simulink model "TPTC_Vehicle_dynamics_pedal2torque_NeglectSOC"  (R2026a)
settings: Solver=ode23tb  StopTime=40
model workspace (MAT data in the model file):
  BattChrgMax = -500000
  BattDischrgMax = 500000
  ChrgLmt_bpt = [1 1 1 1 1 1 1 1 0.7 0.35 0]
  DischrgLmt_bpt = [0 0.35 0.7 1 1 1 1 1 1 1 1]
  SOC_bpt = [0 10 20 30 40 50 60 70 80 90 100]
  motorMaxTorqueNm = [500 500 500 500 500 500 416.666666667 357.142857143 312.5 277.777777778 250 227.272727273 ... (16 elements, 1x16)]
  motorSpeedRadPs = [0 40 80 120 160 200 240 280 320 360 400 440 ... (16 elements, 1x16)]
values from neighbouring files (symbols this model uses):
  alpha_thr = Simulink.Parameter(300)    [init_MCU_ASR_params_only.m]
  eta_drv = Simulink.Parameter(0.95)    [init_MCU_ASR_params_only.m]
  gear_ratio_F = Simulink.Parameter(10.91)    [init_MCU_ASR_params_only.m]
  gear_ratio_R = Simulink.Parameter(11.62)    [init_MCU_ASR_params_only.m]
  J_axle = Simulink.Parameter(2*I_tire)    [init_MCU_ASR_params_only.m]
  Kd_damp = Simulink.Parameter(0.025)    [init_MCU_ASR_params_only.m]
  R_tire = Simulink.Parameter(r)    [init_MCU_ASR_params_only.m]
  T_active = Simulink.Parameter(15)    [init_MCU_ASR_params_only.m]
  T_damp_lim = Simulink.Parameter(18)    [init_MCU_ASR_params_only.m]
  tau_lpf_damp = Simulink.Parameter(0.060)    [init_MCU_ASR_params_only.m]
  Tlim_down_rate = Simulink.Parameter(2000)    [init_MCU_ASR_params_only.m]
  Tlim_up_rate = Simulink.Parameter(120)    [init_MCU_ASR_params_only.m]
  Tlim_warn_rate = Simulink.Parameter(600)    [init_MCU_ASR_params_only.m]
  Tmax_mot = Simulink.Parameter(Tn_motor)    [init_MCU_ASR_params_only.m]
  Ts_asr = Simulink.Parameter(0.001)    [init_MCU_ASR_params_only.m]
undefined symbols (not defined in the file or in its folder): dspblkCoreblockFVToolHelper, gcbh, gear_ratio
libraries: autolibsharedcoupling x8, simulink x3, autolibshareddiff x2, autolibmappedmotor x2, slpidlib x1, autolibdatasheetbattery x1, sim3dlib x1, sim3dautolib x1, vehdynlibsteering x1
(part 3 of 4)

== matlab function TPTC_Vehicle_dynamics_pedal2torque_NeglectSOC/03_MCU_ASR_Controller1/Slip_Detector_Rear/MATLAB Function ==
  data: Te input; risk output; warn output; alpha input; Tload input; omega input; Te_opp input; alpha_opp input; Tload_opp input; omega_opp input; T_active input; state output; alpha_thr input; Ts input; load_ratio output; follow_bad output; axis_diverge output; startup_guard output
function [risk,warn,state,load_ratio,follow_bad,axis_diverge,startup_guard] = f( ...
    Te,alpha,Tload,omega, ...
    Te_opp,alpha_opp,Tload_opp,omega_opp, ...
    T_active,alpha_thr,Ts)
%#codegen

% ============================================================
% MCU级 TCPC/ASR Slip Detector
%
% 核心判据：
% 1. Tload_est / Te 偏低
% 2. Te 增加时，Tload_est 不跟随增加
% 3. alpha 异常升高作为确认条件
%
% axis_diverge 只做诊断输出，不单独触发 warn/risk
%
% state:
%   0 Normal
%   1 Warning
%   2 Risk
% ============================================================

persistent risk_z warn_z
persistent Te_z Tload_z omega_z omega_opp_z
persistent active_cnt risk_enter_cnt warn_enter_cnt risk_exit_cnt warn_exit_cnt

if isempty(risk_z)
    risk_z = false;
    warn_z = false;

    Te_z = 0.0;
    Tload_z = 0.0;
    omega_z = 0.0;
    omega_opp_z = 0.0;

    active_cnt = 0.0;
    risk_enter_cnt = 0.0;
    warn_enter_cnt = 0.0;
    risk_exit_cnt = 0.0;
    warn_exit_cnt = 0.0;
end

% =========================
% 采样时间保护
% =========================
if Ts <= 0.0
    Ts_eff = 1e-3;
else
    Ts_eff = Ts;
end

% =========================
% 可标定参数
% =========================

% 负载比例阈值
k_load_risk = 0.72;
k_load_warn = 0.86;

% 跟随性阈值
k_follow_risk = 0.20;
k_follow_warn = 0.40;

% alpha 阈值
alpha_warn_gain = 0.65;
alpha_risk_gain = 1.00;

% 起步保护
startup_guard_time = 0.30;
startup_guard_steps = ceil(startup_guard_time / Ts_eff);

% 起步阶段只允许较强 risk
alpha_start_risk_gain = 1.40;
k_load_start_risk = 0.55;

% 进入确认时间
% risk 不要太慢，否则压不住滑移；warn 稍微确认
risk_enter_confirm_time = 0.005;  % 5 ms
warn_enter_confirm_time = 0.020;  % 20 ms

risk_enter_steps = ceil(risk_enter_confirm_time / Ts_eff);
warn_enter_steps = ceil(warn_enter_confirm_time / Ts_eff);

% 退出确认时间
risk_exit_confirm_time = 0.080;   % 80 ms，避免频繁退出
warn_exit_confirm_time = 0.050;   % 50 ms

risk_exit_steps = ceil(risk_exit_confirm_time / Ts_eff);
warn_exit_steps = ceil(warn_exit_confirm_time / Ts_eff);

% dTe 太小时不判断跟随性
dTe_min = max(0.02*T_active, 0.5);

% 前后轴分化诊断阈值
alpha_diff_thr = 0.80*alpha_thr;
omega_diff_thr = 5.0;
omega_diff_rate_thr = 50.0;

% =========================
% 有效驱动区
% =========================
active = (Te > T_active);

if active
    active_cnt = active_cnt + 1.0;
else
    active_cnt = 0.0;
end

startup_guard = active && (active_cnt <= startup_guard_steps);

% =========================
% 负载比例
% =========================
Te_eff = max(Te, 1.0);
load_ratio_raw = Tload / Te_eff;

if load_ratio_raw < 0.0
    load_ratio = 0.0;
elseif load_ratio_raw > 2.0
    load_ratio = 2.0;
else
    load_ratio = load_ratio_raw;
end

load_gap_risk = (load_ratio < k_load_risk);
load_gap_warn = (load_ratio < k_load_warn);

% =========================
% Tload 是否随 Te 增加
% =========================
dTe = Te - Te_z;
dTload = Tload - Tload_z;

torque_rising = (dTe > dTe_min);

follow_bad_risk = torque_rising && (dTload < k_follow_risk*dTe);
follow_bad_warn = torque_rising && (dTload < k_follow_warn*dTe);

follow_bad = follow_bad_risk;

% =========================
% alpha 异常
% =========================
alpha_risk = (alpha > alpha_risk_gain*alpha_thr);
alpha_warn = (alpha > alpha_warn_gain*alpha_thr);

% =========================
% 前后轴分化，仅诊断
% =========================
omega_diff = omega - omega_opp;
omega_diff_z = omega_z - omega_opp_z;
d_omega_diff = (omega_diff - omega_diff_z) / Ts_eff;

alpha_diverge = (alpha > alpha_opp + alpha_diff_thr) && alpha_warn;

omega_diverge = (~startup_guard) && ...
                (omega_diff > omega_diff_thr) && ...
                (d_omega_diff > omega_diff_rate_thr);

axis_diverge = alpha_diverge || omega_diverge;

% =========================
% 原始进入判据
% =========================
if startup_guard

    % 起步保护阶段：
    % 不允许 warn，只允许强 risk
    warn_enter_raw = false;

    risk_enter_raw = active && ...
                     (alpha > alpha_start_risk_gain*alpha_thr) && ...
                     ((load_ratio < k_load_start_risk) || follow_bad_risk);

else

    % 正常阶段：
    % axis_diverge 不直接触发
    risk_enter_raw = active && ...
                     alpha_risk && ...
                     (load_gap_risk || follow_bad_risk);

    warn_enter_raw = active && ...
                     alpha_warn && ...
                     (load_gap_warn || follow_bad_warn);
end

% =========================
% 进入确认
% =========================
if risk_enter_raw
    risk_enter_cnt = risk_enter_cnt + 1.0;
else
    risk_enter_cnt = 0.0;
end

if warn_enter_raw
    warn_enter_cnt = warn_enter_cnt + 1.0;
else
    warn_enter_cnt = 0.0;
end

risk_enter = (risk_enter_cnt >= risk_enter_steps);
warn_enter = (warn_enter_cnt >= warn_enter_steps);

% =========================
% 退出判据
% =========================
risk_exit_raw = (~active) || ...
                ( ...
                  (alpha < 0.45*alpha_thr) && ...
                  (load_ratio > 0.88) && ...
                  (~follow_bad_warn) ...
                );

warn_exit_raw = (~active) || ...
                ( ...
                  (alpha < 0.35*alpha_thr) && ...
                  (load_ratio > 0.96) && ...
                  (~follow_bad_warn) ...
                );

if risk_exit_raw
    risk_exit_cnt = risk_exit_cnt + 1.0;
else
    risk_exit_cnt = 0.0;
end

if warn_exit_raw
    warn_exit_cnt = warn_exit_cnt + 1.0;
else
    warn_exit_cnt = 0.0;
end

risk_exit = (risk_exit_cnt >= risk_exit_steps);
warn_exit = (warn_exit_cnt >= warn_exit_steps);

% =========================
% risk 滞回
% =========================
if risk_z
    if risk_exit
        risk_z = false;
        risk_exit_cnt = 0.0;
    end
else
    if risk_enter
        risk_z = true;
        risk_enter_cnt = 0.0;
    end
end

% =========================
% warn 滞回
% =========================
if risk_z
    warn_z = false;
    warn_exit_cnt = 0.0;
else
    if warn_z
        if warn_exit
            warn_z = false;
            warn_exit_cnt = 0.0;
        end
    else
        if warn_enter
            warn_z = true;
            warn_enter_cnt = 0.0;
        end
    end
end

% =========================
% 输出
% =========================
risk = risk_z;
warn = warn_z;

if risk_z
    state = 2.0;
elseif warn_z
    state = 1.0;
else
    state = 0.0;
end

% =========================
% 更新历史量
% =========================
Te_z = Te;
Tload_z = Tload;
omega_z = omega;
omega_opp_z = omega_opp;

end

== matlab function TPTC_Vehicle_dynamics_pedal2torque_NeglectSOC/03_MCU_ASR_Controller1/Torque_Limiter_Front/Fast_Down_Slow_Up_Limiter ==
  data: T_vcu input; Tlim output; risk input; warn input; Tload input; Tmax_mot parameter; state output; Tlim_up_rate parameter; Tlim_down_rate parameter; Tlim_warn_rate parameter; Ts_asr parameter
function [Tlim,state] = f(T_vcu,risk,warn,Tload,Tmax_mot,Tlim_up_rate,Tlim_down_rate,Tlim_warn_rate,Ts_asr)
%#codegen

% ============================================================
% MCU级 TCPC/ASR 限扭器 v5
%
% state:
%   0 Normal
%   1 Warning
%   2 SpinDown
%   3 Hold
%   4 Recovery
%
% 核心策略：
%   1. risk 时快速降低 Tcap 和 Tlim
%   2. 打滑后进入 Hold，不立即恢复
%   3. Recovery 只恢复到 Tcap
%   4. Tcap 只在稳定后小斜率上探
%   5. 避免恢复-打滑-恢复的大幅搏动
% ============================================================

persistent Tlim_z state_z hold_cnt recover_cnt drive_cnt
persistent Tload_lpf_z first_run
persistent Tcap_z stable_cnt

if isempty(Tlim_z)
    Tlim_z = 0.0;
    state_z = 0.0;
    hold_cnt = 0.0;
    recover_cnt = 0.0;
    drive_cnt = 0.0;

    Tload_lpf_z = 0.0;
    first_run = true;

    Tcap_z = 0.0;
    stable_cnt = 0.0;
end

% =========================
% 状态定义
% =========================
S_NORMAL   = 0.0;
S_WARNING  = 1.0;
S_SPINDOWN = 2.0;
S_HOLD     = 3.0;
S_RECOVERY = 4.0;

% =========================
% 采样时间保护
% =========================
if Ts_asr <= 0.0
    Ts = 1e-3;
else
    Ts = Ts_asr;
end

% =========================
% 可标定参数
% =========================

% 状态时间
spin_hold_time = 0.25;        % 低扭矩保持 250 ms
recovery_min_time = 0.35;     % Recovery 至少 350 ms

spin_hold_steps = ceil(spin_hold_time / Ts);
recovery_min_steps = ceil(recovery_min_time / Ts);

% Tload 低通
tau_Tload = 0.060;            % 60 ms

% SpinDown 目标
T_decel_margin = 18.0;        % T_spin_target = Tload_ref - margin
T_spin_min = 0.0;
T_spin_keep_min = 0.0;

% 动态 Tcap
Tcap_margin_recover = 8.0;    % risk 后 Tcap 收敛到 Tload_ref + 8
Tcap_drop_rate = 5000.0;      % risk 时 Tcap 下降速率
Tcap_min = 0.0;

% Tcap 试探增长
Tcap_probe_rate_slow = 6.0;   % 低附着/不确定
Tcap_probe_rate_mid  = 25.0;  % 中等
Tcap_probe_rate_fast = 80.0;  % 高附着确认

stable_time_for_probe = 0.30; % 稳定 300 ms 后才允许 Tcap 上探
stable_steps_for_probe = ceil(stable_time_for_probe / Ts);

% warn 处理
warn_freeze_time = 0.10;      % Recovery 中 warn 冻结 100 ms
T_warn_min = 15.0;

% 上升速率
Tlim_normal_up_rate = 1.2*Tlim_up_rate;
Tlim_recovery_up_rate = 0.45*Tlim_up_rate;

% 起步软限制
startup_time = 0.60;
startup_steps = ceil(startup_time / Ts);
T_cmd_active_thr = max(1.0,0.02*Tmax_mot);
startup_ramp_rate = 0.40*Tmax_mot / max(startup_time,Ts);

% 最终输出斜率保护
Tlim_final_down_rate = max(Tlim_down_rate,1500.0);
Tlim_final_up_rate   = max(Tlim_recovery_up_rate,1.0);

% =========================
% 目标扭矩
% =========================
target_raw = min(max(T_vcu,0.0),Tmax_mot);

if first_run
    Tlim_z = 0.0;
    Tload_lpf_z = max(Tload,0.0);
    Tcap_z = target_raw;
    first_run = false;
end

% =========================
% 驱动计时
% =========================
cmd_active = target_raw > T_cmd_active_thr;

if cmd_active
    drive_cnt = drive_cnt + 1.0;
else
    drive_cnt = 0.0;
end

startup_phase = cmd_active && (drive_cnt <= startup_steps);

% =========================
% Tload 低通
% =========================
Tload_eff = Tload;

if Tload_eff < 0.0
    Tload_eff = 0.0;
end

a_lpf = Ts / (tau_Tload + Ts);
Tload_lpf_z = Tload_lpf_z + a_lpf*(Tload_eff - Tload_lpf_z);

Tload_ref = Tload_lpf_z;

% =========================
% Tcap 更新
% =========================

% 当前负载跟随程度
Tlim_eff = max(Tlim_z,1.0);
load_ratio_cap = Tload_ref / Tlim_eff;

load_follow_good = (load_ratio_cap > 0.90);
load_follow_mid  = (load_ratio_cap > 0.75);

if risk

    % risk 时快速压低 Tcap
    Tcap_target_down = Tload_ref + Tcap_margin_recover;

    if Tcap_target_down < Tcap_min
        Tcap_target_down = Tcap_min;
    end

    if Tcap_z > Tcap_target_down
        Tcap_z = Tcap_z - Tcap_drop_rate*Ts;

        if Tcap_z < Tcap_target_down
            Tcap_z = Tcap_target_down;
        end
    else
        Tcap_z = Tcap_target_down;
    end

    stable_cnt = 0.0;

else

    if ~warn
        stable_cnt = stable_cnt + 1.0;
    else
        stable_cnt = 0.0;
    end

    if stable_cnt >= stable_steps_for_probe

        if load_follow_good
            Tcap_probe_rate_now = Tcap_probe_rate_fast;
        elseif load_follow_mid
            Tcap_probe_rate_now = Tcap_probe_rate_mid;
        else
            Tcap_probe_rate_now = Tcap_probe_rate_slow;
        end

        if Tcap_z < target_raw
            Tcap_z = Tcap_z + Tcap_probe_rate_now*Ts;

            if Tcap_z > target_raw
                Tcap_z = target_raw;
            end
        else
            Tcap_z = target_raw;
        end
    end
end

% Tcap 限幅
if Tcap_z > Tmax_mot
    Tcap_z = Tmax_mot;
elseif Tcap_z < 0.0
    Tcap_z = 0.0;
end

% 实际目标被 Tcap 限制
target = min(target_raw,Tcap_z);

% VCU 请求降低时，立即跟随
if Tlim_z > target_raw
    Tlim_z = target_raw;
end

% =========================
% SpinDown 目标
% =========================
T_spin_target = Tload_ref - T_decel_margin;

if T_spin_target < T_spin_min
    T_spin_target = T_spin_min;
end

if T_spin_target > target_raw
    T_spin_target = target_raw;
end

T_spin_keep_eff = min(T_spin_keep_min,target_raw);
T_warn_min_eff = min(T_warn_min,target_raw);

% =========================
% 状态转移
% =========================
switch state_z

    case S_NORMAL

        hold_cnt = 0.0;
        recover_cnt = 0.0;

        if risk
            state_z = S_SPINDOWN;
            hold_cnt = spin_hold_steps;

        elseif warn
            state_z = S_WARNING;

        else
            state_z = S_NORMAL;
        end

    case S_WARNING

        if risk
            state_z = S_SPINDOWN;
            hold_cnt = spin_hold_steps;

        elseif warn
            state_z = S_WARNING;

        else
            if Tlim_z < target
                state_z = S_RECOVERY;
                recover_cnt = recovery_min_steps;
            else
                state_z = S_NORMAL;
            end
        end

    case S_SPINDOWN

        if risk
            state_z = S_SPINDOWN;
            hold_cnt = spin_hold_steps;
        else
            state_z = S_HOLD;
            hold_cnt = spin_hold_steps;
        end

    case S_HOLD

        if risk
            state_z = S_SPINDOWN;
            hold_cnt = spin_hold_steps;
        else
            if hold_cnt > 0.0
                hold_cnt = hold_cnt - 1.0;
                state_z = S_HOLD;
            else
                state_z = S_RECOVERY;
                recover_cnt = recovery_min_steps;
            end
        end

    case S_RECOVERY

        if risk
            state_z = S_SPINDOWN;
            hold_cnt = spin_hold_steps;

        elseif warn
            % warn 时只冻结，不强降
            state_z = S_HOLD;
            hold_cnt = ceil(warn_freeze_time / Ts);

        else
            if recover_cnt > 0.0
                recover_cnt = recover_cnt - 1.0;
                state_z = S_RECOVERY;
            else
                if Tlim_z < target
                    state_z = S_RECOVERY;
                else
                    state_z = S_NORMAL;
                    recover_cnt = 0.0;
                end
            end
        end

    otherwise

        state_z = S_NORMAL;
        hold_cnt = 0.0;
        recover_cnt = 0.0;
end

% =========================
% 计算 Tlim_ref
% =========================
Tlim_ref = Tlim_z;

if state_z == S_SPINDOWN

    % 快速降到 Tload_ref - margin
    if Tlim_z > T_spin_target
        Tlim_ref = Tlim_z - Tlim_down_rate*Ts;

        if Tlim_ref < T_spin_target
            Tlim_ref = T_spin_target;
        end
    else
        Tlim_ref = Tlim_z;
    end

    if Tlim_ref < T_spin_keep_eff
        Tlim_ref = T_spin_keep_eff;
    end

elseif state_z == S_HOLD

    % Hold：保持低扭矩；如果仍偏高，继续缓慢向 T_spin_target 靠近
    if Tlim_z > T_spin_target
        Tlim_ref = Tlim_z - 0.20*Tlim_down_rate*Ts;

        if Tlim_ref < T_spin_target
            Tlim_ref = T_spin_target;
        end
    else
        Tlim_ref = Tlim_z;
    end

    if Tlim_ref < T_spin_keep_eff
        Tlim_ref = T_spin_keep_eff;
    end

elseif state_z == S_WARNING

    % Warning：只轻微降扭
    Tlim_ref = Tlim_z - Tlim_warn_rate*Ts;

    if Tlim_ref < T_warn_min_eff
        Tlim_ref = T_warn_min_eff;
    end

    if Tlim_ref > target
        Tlim_ref = target;
    end

elseif state_z == S_RECOVERY

    % Recovery：只恢复到 target = min(T_vcu, Tcap)
    if target > Tlim_z
        Tlim_ref = Tlim_z + Tlim_recovery_up_rate*Ts;

        if Tlim_ref > target
            Tlim_ref = target;
        end
    else
        Tlim_ref = target;
    end

else

    % Normal：也只跟随 target = min(T_vcu, Tcap)
    if target > Tlim_z
        Tlim_ref = Tlim_z + Tlim_normal_up_rate*Ts;

        if Tlim_ref > target
            Tlim_ref = target;
        end
    else
        Tlim_ref = target;
    end
end

% =========================
% 起步软限制
% =========================
if startup_phase && ...
   (state_z == S_NORMAL || state_z == S_WARNING || state_z == S_RECOVERY)

    startup_Tlim = startup_ramp_rate * drive_cnt * Ts;

    if Tlim_ref > startup_Tlim
        Tlim_ref = startup_Tlim;
    end
end

% =========================
% 最终输出斜率保护
% =========================
dT = Tlim_ref - Tlim_z;

if dT > Tlim_final_up_rate*Ts
    dT = Tlim_final_up_rate*Ts;
elseif dT < -Tlim_final_down_rate*Ts
    dT = -Tlim_final_down_rate*Ts;
end

Tlim_z = Tlim_z + dT;

% =========================
% 最终限幅
% =========================
if Tlim_z > Tmax_mot
    Tlim_z = Tmax_mot;
elseif Tlim_z < 0.0
    Tlim_z = 0.0;
end

if Tlim_z > target_raw
    Tlim_z = target_raw;
end

Tlim = Tlim_z;
state = state_z;

end

== matlab function TPTC_Vehicle_dynamics_pedal2torque_NeglectSOC/03_MCU_ASR_Controller1/Torque_Limiter_Rear/Fast_Down_Slow_Up_Limiter ==
  data: T_vcu input; Tlim output; risk input; warn input; Tload input; state output; Tmax_mot parameter; Tlim_up_rate parameter; Tlim_down_rate parameter; Tlim_warn_rate parameter; Ts_asr parameter
function [Tlim,state] = f(T_vcu,risk,warn,Tload,Tmax_mot,Tlim_up_rate,Tlim_down_rate,Tlim_warn_rate,Ts_asr)
%#codegen

% ============================================================
% MCU级 TCPC/ASR 限扭器 v5
%
% state:
%   0 Normal
%   1 Warning
%   2 SpinDown
%   3 Hold
%   4 Recovery
%
% 核心策略：
%   1. risk 时快速降低 Tcap 和 Tlim
%   2. 打滑后进入 Hold，不立即恢复
%   3. Recovery 只恢复到 Tcap
%   4. Tcap 只在稳定后小斜率上探
%   5. 避免恢复-打滑-恢复的大幅搏动
% ============================================================

persistent Tlim_z state_z hold_cnt recover_cnt drive_cnt
persistent Tload_lpf_z first_run
persistent Tcap_z stable_cnt

if isempty(Tlim_z)
    Tlim_z = 0.0;
    state_z = 0.0;
    hold_cnt = 0.0;
    recover_cnt = 0.0;
    drive_cnt = 0.0;

    Tload_lpf_z = 0.0;
    first_run = true;

    Tcap_z = 0.0;
    stable_cnt = 0.0;
end

% =========================
% 状态定义
% =========================
S_NORMAL   = 0.0;
S_WARNING  = 1.0;
S_SPINDOWN = 2.0;
S_HOLD     = 3.0;
S_RECOVERY = 4.0;

% =========================
% 采样时间保护
% =========================
if Ts_asr <= 0.0
    Ts = 1e-3;
else
    Ts = Ts_asr;
end

% =========================
% 可标定参数
% =========================

% 状态时间
spin_hold_time = 0.25;        % 低扭矩保持 250 ms
recovery_min_time = 0.35;     % Recovery 至少 350 ms

spin_hold_steps = ceil(spin_hold_time / Ts);
recovery_min_steps = ceil(recovery_min_time / Ts);

% Tload 低通
tau_Tload = 0.060;            % 60 ms

% SpinDown 目标
T_decel_margin = 18.0;        % T_spin_target = Tload_ref - margin
T_spin_min = 0.0;
T_spin_keep_min = 0.0;

% 动态 Tcap
Tcap_margin_recover = 8.0;    % risk 后 Tcap 收敛到 Tload_ref + 8
Tcap_drop_rate = 5000.0;      % risk 时 Tcap 下降速率
Tcap_min = 0.0;

% Tcap 试探增长
Tcap_probe_rate_slow = 6.0;   % 低附着/不确定
Tcap_probe_rate_mid  = 25.0;  % 中等
Tcap_probe_rate_fast = 80.0;  % 高附着确认

stable_time_for_probe = 0.30; % 稳定 300 ms 后才允许 Tcap 上探
stable_steps_for_probe = ceil(stable_time_for_probe / Ts);

% warn 处理
warn_freeze_time = 0.10;      % Recovery 中 warn 冻结 100 ms
T_warn_min = 15.0;

% 上升速率
Tlim_normal_up_rate = 1.2*Tlim_up_rate;
Tlim_recovery_up_rate = 0.45*Tlim_up_rate;

% 起步软限制
startup_time = 0.60;
startup_steps = ceil(startup_time / Ts);
T_cmd_active_thr = max(1.0,0.02*Tmax_mot);
startup_ramp_rate = 0.40*Tmax_mot / max(startup_time,Ts);

% 最终输出斜率保护
Tlim_final_down_rate = max(Tlim_down_rate,1500.0);
Tlim_final_up_rate   = max(Tlim_recovery_up_rate,1.0);

% =========================
% 目标扭矩
% =========================
target_raw = min(max(T_vcu,0.0),Tmax_mot);

if first_run
    Tlim_z = 0.0;
    Tload_lpf_z = max(Tload,0.0);
    Tcap_z = target_raw;
    first_run = false;
end

% =========================
% 驱动计时
% =========================
cmd_active = target_raw > T_cmd_active_thr;

if cmd_active
    drive_cnt = drive_cnt + 1.0;
else
    drive_cnt = 0.0;
end

startup_phase = cmd_active && (drive_cnt <= startup_steps);

% =========================
% Tload 低通
% =========================
Tload_eff = Tload;

if Tload_eff < 0.0
    Tload_eff = 0.0;
end

a_lpf = Ts / (tau_Tload + Ts);
Tload_lpf_z = Tload_lpf_z + a_lpf*(Tload_eff - Tload_lpf_z);

Tload_ref = Tload_lpf_z;

% =========================
% Tcap 更新
% =========================

% 当前负载跟随程度
Tlim_eff = max(Tlim_z,1.0);
load_ratio_cap = Tload_ref / Tlim_eff;

load_follow_good = (load_ratio_cap > 0.90);
load_follow_mid  = (load_ratio_cap > 0.75);

if risk

    % risk 时快速压低 Tcap
    Tcap_target_down = Tload_ref + Tcap_margin_recover;

    if Tcap_target_down < Tcap_min
        Tcap_target_down = Tcap_min;
    end

    if Tcap_z > Tcap_target_down
        Tcap_z = Tcap_z - Tcap_drop_rate*Ts;

        if Tcap_z < Tcap_target_down
            Tcap_z = Tcap_target_down;
        end
    else
        Tcap_z = Tcap_target_down;
    end

    stable_cnt = 0.0;

else

    if ~warn
        stable_cnt = stable_cnt + 1.0;
    else
        stable_cnt = 0.0;
    end

    if stable_cnt >= stable_steps_for_probe

        if load_follow_good
            Tcap_probe_rate_now = Tcap_probe_rate_fast;
        elseif load_follow_mid
            Tcap_probe_rate_now = Tcap_probe_rate_mid;
        else
            Tcap_probe_rate_now = Tcap_probe_rate_slow;
        end

        if Tcap_z < target_raw
            Tcap_z = Tcap_z + Tcap_probe_rate_now*Ts;

            if Tcap_z > target_raw
                Tcap_z = target_raw;
            end
        else
            Tcap_z = target_raw;
        end
    end
end

% Tcap 限幅
if Tcap_z > Tmax_mot
    Tcap_z = Tmax_mot;
elseif Tcap_z < 0.0
    Tcap_z = 0.0;
end

% 实际目标被 Tcap 限制
target = min(target_raw,Tcap_z);

% VCU 请求降低时，立即跟随
if Tlim_z > target_raw
    Tlim_z = target_raw;
end

% =========================
% SpinDown 目标
% =========================
T_spin_target = Tload_ref - T_decel_margin;

if T_spin_target < T_spin_min
    T_spin_target = T_spin_min;
end

if T_spin_target > target_raw
    T_spin_target = target_raw;
end

T_spin_keep_eff = min(T_spin_keep_min,target_raw);
T_warn_min_eff = min(T_warn_min,target_raw);

% =========================
% 状态转移
% =========================
switch state_z

    case S_NORMAL

        hold_cnt = 0.0;
        recover_cnt = 0.0;

        if risk
            state_z = S_SPINDOWN;
            hold_cnt = spin_hold_steps;

        elseif warn
            state_z = S_WARNING;

        else
            state_z = S_NORMAL;
        end

    case S_WARNING

        if risk
            state_z = S_SPINDOWN;
            hold_cnt = spin_hold_steps;

        elseif warn
            state_z = S_WARNING;

        else
            if Tlim_z < target
                state_z = S_RECOVERY;
                recover_cnt = recovery_min_steps;
            else
                state_z = S_NORMAL;
            end
        end

    case S_SPINDOWN

        if risk
            state_z = S_SPINDOWN;
            hold_cnt = spin_hold_steps;
        else
            state_z = S_HOLD;
            hold_cnt = spin_hold_steps;
        end

    case S_HOLD

        if risk
            state_z = S_SPINDOWN;
            hold_cnt = spin_hold_steps;
        else
            if hold_cnt > 0.0
                hold_cnt = hold_cnt - 1.0;
                state_z = S_HOLD;
            else
                state_z = S_RECOVERY;
                recover_cnt = recovery_min_steps;
            end
        end

    case S_RECOVERY

        if risk
            state_z = S_SPINDOWN;
            hold_cnt = spin_hold_steps;

        elseif warn
            % warn 时只冻结，不强降
            state_z = S_HOLD;
            hold_cnt = ceil(warn_freeze_time / Ts);

        else
            if recover_cnt > 0.0
                recover_cnt = recover_cnt - 1.0;
                state_z = S_RECOVERY;
            else
                if Tlim_z < target
                    state_z = S_RECOVERY;
                else
                    state_z = S_NORMAL;
                    recover_cnt = 0.0;
                end
            end
        end

    otherwise

        state_z = S_NORMAL;
        hold_cnt = 0.0;
        recover_cnt = 0.0;
end

% =========================
% 计算 Tlim_ref
% =========================
Tlim_ref = Tlim_z;

if state_z == S_SPINDOWN

    % 快速降到 Tload_ref - margin
    if Tlim_z > T_spin_target
        Tlim_ref = Tlim_z - Tlim_down_rate*Ts;

        if Tlim_ref < T_spin_target
            Tlim_ref = T_spin_target;
        end
    else
        Tlim_ref = Tlim_z;
    end

    if Tlim_ref < T_spin_keep_eff
        Tlim_ref = T_spin_keep_eff;
    end

elseif state_z == S_HOLD

    % Hold：保持低扭矩；如果仍偏高，继续缓慢向 T_spin_target 靠近
    if Tlim_z > T_spin_target
        Tlim_ref = Tlim_z - 0.20*Tlim_down_rate*Ts;

        if Tlim_ref < T_spin_target
            Tlim_ref = T_spin_target;
        end
    else
        Tlim_ref = Tlim_z;
    end

    if Tlim_ref < T_spin_keep_eff
        Tlim_ref = T_spin_keep_eff;
    end

elseif state_z == S_WARNING

    % Warning：只轻微降扭
    Tlim_ref = Tlim_z - Tlim_warn_rate*Ts;

    if Tlim_ref < T_warn_min_eff
        Tlim_ref = T_warn_min_eff;
    end

    if Tlim_ref > target
        Tlim_ref = target;
    end

elseif state_z == S_RECOVERY

    % Recovery：只恢复到 target = min(T_vcu, Tcap)
    if target > Tlim_z
        Tlim_ref = Tlim_z + Tlim_recovery_up_rate*Ts;

        if Tlim_ref > target
            Tlim_ref = target;
        end
    else
        Tlim_ref = target;
    end

else

    % Normal：也只跟随 target = min(T_vcu, Tcap)
    if target > Tlim_z
        Tlim_ref = Tlim_z + Tlim_normal_up_rate*Ts;

        if Tlim_ref > target
            Tlim_ref = target;
        end
    else
        Tlim_ref = target;
    end
end

% =========================
% 起步软限制
% =========================
if startup_phase && ...
   (state_z == S_NORMAL || state_z == S_WARNING || state_z == S_RECOVERY)

    startup_Tlim = startup_ramp_rate * drive_cnt * Ts;

    if Tlim_ref > startup_Tlim
        Tlim_ref = startup_Tlim;
    end
end

% =========================
% 最终输出斜率保护
% =========================
dT = Tlim_ref - Tlim_z;

if dT > Tlim_final_up_rate*Ts
    dT = Tlim_final_up_rate*Ts;
elseif dT < -Tlim_final_down_rate*Ts
    dT = -Tlim_final_down_rate*Ts;
end

Tlim_z = Tlim_z + dT;

% =========================
% 最终限幅
% =========================
if Tlim_z > Tmax_mot
    Tlim_z = Tmax_mot;
elseif Tlim_z < 0.0
    Tlim_z = 0.0;
end

if Tlim_z > target_raw
    Tlim_z = target_raw;
end

Tlim = Tlim_z;
state = state_z;

end

== matlab function TPTC_Vehicle_dynamics_pedal2torque_NeglectSOC/Environment/Fast_Down_Slow_Up_Limiter ==
  data: miu_in input; time input; miu output
function miu = f(miu_in, time)
    if time > 10
        % 当时间大于20秒时，miu等于原值乘以0.5
        miu = miu_in ;  
    elseif time > 5
        % 当时间大于10秒（且不超过20秒）时，miu等于原值
        miu = miu_in*0.3;        
    else
        % 当时间不大于10秒时，赋予默认值0（可根据你的实际需求修改）
        miu = miu_in;             
    end
end

== matlab function TPTC_Vehicle_dynamics_pedal2torque_NeglectSOC/Powertrain/03_MCU_TPTC_Controller/Slip_Detector_Front/MATLAB Function1 ==
  data: Te input; risk output; warn output; alpha input; Tload input; omega input; Te_opp input; alpha_opp input; Tload_opp input; omega_opp input; T_active input; state output; alpha_thr input; Ts input; load_ratio output; follow_bad output; axis_diverge output; startup_guard output; Treq input; limit_ratio output
function [risk,warn,state,load_ratio,follow_bad,...
    axis_diverge,startup_guard,limit_ratio] = f( ...
    Te,alpha,Tload,omega, ...
    Te_opp,alpha_opp,Tload_opp,omega_opp, ...
    T_active,alpha_thr,Ts,Treq)
%#codegen

% ============================================================
% MCU级 TPTC/ASR 滑移风险检测状态机
%
% 不使用滑移率，不使用车辆纵向速度。
%
% 输入：
%   Te          本轴实际/估算电机扭矩，N*m
%   alpha       本轴电机机械角加速度，rad/s^2
%   Tload       本轴电机侧负载转矩观测值，N*m
%   omega       本轴电机机械角速度，rad/s
%
%   Te_opp      对轴电机扭矩，N*m
%   alpha_opp   对轴电机角加速度，rad/s^2
%   Tload_opp   对轴负载转矩观测值，N*m
%   omega_opp   对轴电机机械角速度，rad/s
%
%   T_active    有效驱动请求阈值，N*m
%   alpha_thr   基础角加速度阈值，rad/s^2
%   Ts          控制周期，s
%   Treq        限扭前VCU目标扭矩，N*m
%
% 输出：
%   risk           Risk标志
%   warn           Warning标志
%   state          0 Normal / 1 Warning / 2 Risk
%   load_ratio     当前负载支持能力，正常约为1
%   follow_bad     负载传递异常
%   axis_diverge   前后轴动态分化诊断
%   startup_guard  起步保护标志
%   limit_ratio    目标限扭比例
%
% 状态控制：
%   Normal  ：limit_ratio = 1.00
%   Warning ：limit_ratio = 0.82
%   Risk    ：limit_ratio = 0.50~0.70，自适应
%
% 关键修改：
%   1. 持续严重负载缺失可以直接进入Risk；
%   2. 不再强制要求Risk必须伴随明显alpha异常；
%   3. Warning状态真正执行82%轻度限扭；
%   4. Warning期间负载能力仍严重不足时升级Risk；
%   5. Risk/Warning期间冻结正常负载基线；
%   6. 进入和退出均设置计数确认，避免抖振。
% ============================================================


%% ============================================================
% 1. 持久变量
% =============================================================

persistent initialized
persistent state_z

persistent active_cnt
persistent baseline_cnt
persistent baseline_valid
persistent cooldown_cnt

persistent q_fast_z
persistent q_ref_z
persistent q_rate_z

persistent omega_z
persistent omega_opp_z

persistent risk_enter_cnt
persistent warn_enter_cnt
persistent risk_reenter_cnt
persistent severe_load_cnt

persistent state_hold_cnt
persistent stable_cnt

persistent risk_ratio_z


%% ============================================================
% 2. 初始化
% =============================================================

if isempty(initialized)

    state_z = 0.0;

    active_cnt = 0.0;
    baseline_cnt = 0.0;
    baseline_valid = false;
    cooldown_cnt = 0.0;

    q_fast_z = 0.0;
    q_ref_z = 0.0;
    q_rate_z = 0.0;

    omega_z = 0.0;
    omega_opp_z = 0.0;

    risk_enter_cnt = 0.0;
    warn_enter_cnt = 0.0;
    risk_reenter_cnt = 0.0;
    severe_load_cnt = 0.0;

    state_hold_cnt = 0.0;
    stable_cnt = 0.0;

    risk_ratio_z = 0.60;

    initialized = true;
end


%% ============================================================
% 3. 采样周期和输入保护
% =============================================================

if Ts > 0.0
    Ts_eff = Ts;
else
    Ts_eff = 1.0e-3;
end

T_active_eff = max(abs(T_active),1.0);
alpha_thr_eff = max(abs(alpha_thr),1.0);

Treq_abs = abs(Treq);
Te_abs = abs(Te);
Tload_abs = abs(Tload);


%% ============================================================
% 4. 统一角加速度方向
%
% alpha_drv > 0表示电机转速幅值增加。
% =============================================================

drive_dir = 1.0;

if abs(omega) > 1.0

    if omega < 0.0
        drive_dir = -1.0;
    end

elseif Te_abs > 1.0

    if Te < 0.0
        drive_dir = -1.0;
    end
end

alpha_drv = drive_dir*alpha;


drive_dir_opp = 1.0;

if abs(omega_opp) > 1.0

    if omega_opp < 0.0
        drive_dir_opp = -1.0;
    end

elseif abs(Te_opp) > 1.0

    if Te_opp < 0.0
        drive_dir_opp = -1.0;
    end
end

alpha_opp_drv = drive_dir_opp*alpha_opp;


%% ============================================================
% 5. 标定参数
% =============================================================

% 起步保护
startup_guard_time = 0.050;
initial_blank_time = 0.050;

startup_guard_steps = ...
    max(1.0,ceil(startup_guard_time/Ts_eff));

initial_blank_steps = ...
    max(1.0,ceil(initial_blank_time/Ts_eff));


% 正常负载基线学习时间
baseline_learn_time = 0.400;

baseline_learn_steps = ...
    max(1.0,ceil(baseline_learn_time/Ts_eff));


% 回到Normal后的检测冷却时间
cooldown_time = 0.300;

cooldown_steps = ...
    max(1.0,ceil(cooldown_time/Ts_eff));


% Normal状态进入确认
risk_enter_time = 0.008;
warn_enter_time = 0.020;

risk_enter_steps = ...
    max(1.0,ceil(risk_enter_time/Ts_eff));

warn_enter_steps = ...
    max(1.0,ceil(warn_enter_time/Ts_eff));


% Warning重新升级Risk确认
risk_reenter_time = 0.020;

risk_reenter_steps = ...
    max(1.0,ceil(risk_reenter_time/Ts_eff));


% 持续严重负载不足确认
severe_load_time = 0.030;

severe_load_steps = ...
    max(1.0,ceil(severe_load_time/Ts_eff));


% Risk保持和退出确认
risk_hold_time = 0.250;
risk_stable_time = 0.200;

risk_hold_steps = ...
    max(1.0,ceil(risk_hold_time/Ts_eff));

risk_stable_steps = ...
    max(1.0,ceil(risk_stable_time/Ts_eff));


% Warning保持和退出确认
warn_hold_time = 0.300;
warn_stable_time = 0.300;

warn_hold_steps = ...
    max(1.0,ceil(warn_hold_time/Ts_eff));

warn_stable_steps = ...
    max(1.0,ceil(warn_stable_time/Ts_eff));


% 负载指标滤波
tau_q_fast = 0.030;
tau_q_ref = 1.500;
tau_q_rate = 0.030;

a_q_fast = ...
    Ts_eff/(tau_q_fast + Ts_eff);

a_q_ref = ...
    Ts_eff/(tau_q_ref + Ts_eff);

a_q_rate = ...
    Ts_eff/(tau_q_rate + Ts_eff);


% Normal状态负载阈值
q_warn_thr = 0.85;
q_risk_thr = 0.68;
q_dynamic_thr = 0.78;

% 严重负载支持能力阈值
severe_load_thr = 0.72;

% 相对负载下降速率阈值，单位1/s
q_rate_warn_thr = -0.30;
q_rate_risk_thr = -0.70;


% Risk恢复到Warning
support_risk_recover_thr = 0.80;

% Warning恢复期间重新恶化
support_reenter_thr = 0.72;

% Warning退出到Normal
support_normal_thr = 0.88;


% 角加速度阈值
alpha_warn_thr = 0.55*alpha_thr_eff;
alpha_risk_thr = 0.85*alpha_thr_eff;
alpha_strong_thr = 1.25*alpha_thr_eff;


% 限扭比例
warning_limit_ratio = 0.82;

risk_ratio_min = 0.50;
risk_ratio_max = 0.70;
risk_ratio_margin = 0.10;


% 前后轴分化阈值，仅作诊断
alpha_diff_thr = 0.60*alpha_thr_eff;
omega_diff_thr = 10.0;
omega_diff_rate_thr = 80.0;


%% ============================================================
% 6. 有效驱动请求判断
%
% 必须使用限扭前Treq。
% =============================================================

active = (Treq_abs > T_active_eff);

if active

    active_cnt = active_cnt + 1.0;

else

    active_cnt = 0.0;

    state_z = 0.0;

    baseline_cnt = 0.0;
    baseline_valid = false;
    cooldown_cnt = 0.0;

    risk_enter_cnt = 0.0;
    warn_enter_cnt = 0.0;
    risk_reenter_cnt = 0.0;
    severe_load_cnt = 0.0;

    state_hold_cnt = 0.0;
    stable_cnt = 0.0;

    risk_ratio_z = 0.60;
end

startup_guard = ...
    active && (active_cnt <= startup_guard_steps);

initial_blank = ...
    active && (active_cnt <= initial_blank_steps);


%% ============================================================
% 7. 实际扭矩执行比例
% =============================================================

if Treq_abs > 1.0

    torque_ratio_applied = ...
        Te_abs/Treq_abs;

else

    torque_ratio_applied = 0.0;
end

if torque_ratio_applied < 0.0

    torque_ratio_applied = 0.0;

elseif torque_ratio_applied > 1.20

    torque_ratio_applied = 1.20;
end


%% ============================================================
% 8. 负载观测有效性
% =============================================================

observer_valid = ...
    active && ...
    (Te_abs > max(0.20*Treq_abs,...
                  0.50*T_active_eff));


%% ============================================================
% 9. 负载指标
%
% q = |Tload_hat|/|Treq|
%
% 使用限扭前请求作分母，避免限扭动作直接改变分母。
% =============================================================

q_raw = ...
    Tload_abs/max(Treq_abs,1.0);

if q_raw < 0.0

    q_raw = 0.0;

elseif q_raw > 2.50

    q_raw = 2.50;
end


%% ============================================================
% 10. 当前负载快速滤波及变化率
% =============================================================

if ~active

    q_fast_z = q_raw;
    q_ref_z = q_raw;
    q_rate_z = 0.0;

elseif observer_valid

    if active_cnt <= 1.0

        q_fast_z = q_raw;
        q_ref_z = q_raw;
        q_rate_z = 0.0;

    else

        q_fast_old = q_fast_z;

        q_fast_z = ...
            q_fast_z + ...
            a_q_fast*(q_raw-q_fast_z);

        q_rate_raw = ...
            (q_fast_z-q_fast_old)/Ts_eff;

        q_rate_z = ...
            q_rate_z + ...
            a_q_rate*(q_rate_raw-q_rate_z);
    end

else

    % 观测无效时，变化率缓慢回零
    q_rate_z = ...
        q_rate_z + ...
        a_q_rate*(0.0-q_rate_z);
end


%% ============================================================
% 11. 冷却计数
% =============================================================

if cooldown_cnt > 0.0
    cooldown_cnt = cooldown_cnt-1.0;
end


%% ============================================================
% 12. 正常负载基线学习
%
% 只允许在：
%   Normal、基本全扭矩、动态稳定时更新。
% Warning/Risk期间冻结。
% =============================================================

normal_baseline_condition = ...
    active && ...
    observer_valid && ...
    (state_z == 0.0) && ...
    (torque_ratio_applied > 0.92) && ...
    (abs(alpha_drv) < 0.35*alpha_thr_eff);


if normal_baseline_condition

    if ~baseline_valid

        baseline_cnt = baseline_cnt + 1.0;

        if baseline_cnt <= 1.0

            q_ref_z = q_fast_z;

        else

            q_ref_z = ...
                q_ref_z + ...
                a_q_ref*(q_fast_z-q_ref_z);
        end

        if baseline_cnt >= baseline_learn_steps
            baseline_valid = true;
        end

    else

        q_ref_pre = max(q_ref_z,0.02);

        q_full_pre = ...
            q_fast_z/q_ref_pre;

        q_rate_pre = ...
            q_rate_z/q_ref_pre;

        normal_for_update = ...
            (q_full_pre > 0.90) && ...
            (q_full_pre < 1.12) && ...
            (abs(q_rate_pre) < 0.12);

        if normal_for_update

            q_ref_z = ...
                q_ref_z + ...
                a_q_ref*(q_fast_z-q_ref_z);
        end
    end
end


%% ============================================================
% 13. 负载能力指标
%
% q_full：
%   当前负载相对全扭矩正常基线的比例。
%
% q_support：
%   对当前限扭比例补偿后的负载支持能力。
% =============================================================

if baseline_valid

    q_ref_den = max(q_ref_z,0.02);

    q_full = ...
        q_fast_z/q_ref_den;

    q_rate_rel = ...
        q_rate_z/q_ref_den;

    applied_ratio_den = ...
        max(torque_ratio_applied,0.20);

    q_support = ...
        q_fast_z/...
        (q_ref_den*applied_ratio_den);

else

    q_full = 1.0;
    q_rate_rel = 0.0;
    q_support = 1.0;
end


if q_full < 0.0

    q_full = 0.0;

elseif q_full > 3.0

    q_full = 3.0;
end


if q_support < 0.0

    q_support = 0.0;

elseif q_support > 3.0

    q_support = 3.0;
end


% 对外输出当前扭矩水平下的负载支持能力
load_ratio = q_support;


%% ============================================================
% 14. Normal状态检测器使能
% =============================================================

detector_armed = ...
    baseline_valid && ...
    active && ...
    (state_z == 0.0) && ...
    (cooldown_cnt <= 0.0) && ...
    (torque_ratio_applied > 0.90);


%% ============================================================
% 15. 一般负载异常判据
% =============================================================

load_low_warn = ...
    detector_armed && ...
    (q_full < q_warn_thr);

load_low_risk = ...
    detector_armed && ...
    (q_full < q_risk_thr);

load_drop_warn = ...
    detector_armed && ...
    (q_rate_rel < q_rate_warn_thr);

load_drop_risk = ...
    detector_armed && ...
    (q_rate_rel < q_rate_risk_thr);


%% ============================================================
% 16. 持续严重负载能力不足
%
% Normal使用q_full。
% Warning使用补偿限扭影响后的q_support。
%
% 该路径不强制要求alpha异常，用于解决：
% 开式差速器单轮空转被电机平均转速掩盖的问题。
% =============================================================

if state_z == 0.0

    severe_load_metric = q_full;

    severe_load_enable = ...
        detector_armed && ...
        (torque_ratio_applied > 0.90);

elseif state_z == 1.0

    severe_load_metric = q_support;

    severe_load_enable = ...
        active && ...
        observer_valid && ...
        (torque_ratio_applied > 0.50);

else

    severe_load_metric = q_support;
    severe_load_enable = false;
end


severe_load_raw = ...
    severe_load_enable && ...
    (severe_load_metric < severe_load_thr);


if severe_load_raw

    severe_load_cnt = severe_load_cnt + 1.0;

    if severe_load_cnt > severe_load_steps
        severe_load_cnt = severe_load_steps;
    end

else

    severe_load_cnt = 0.0;
end


severe_load_confirmed = ...
    (severe_load_cnt >= severe_load_steps);


follow_bad = ...
    load_low_warn || ...
    load_drop_warn || ...
    severe_load_confirmed || ...
    ( ...
      (state_z ~= 0.0) && ...
      (q_support < support_risk_recover_thr) ...
    );


%% ============================================================
% 17. 电机角加速度条件
% =============================================================

alpha_warn = ...
    (alpha_drv > alpha_warn_thr);

alpha_risk = ...
    (alpha_drv > alpha_risk_thr);

alpha_strong = ...
    (alpha_drv > alpha_strong_thr);


%% ============================================================
% 18. 前后轴动态分化诊断
%
% 当前仅输出诊断，不直接决定状态。
% =============================================================

omega_diff = ...
    abs(omega)-abs(omega_opp);

omega_diff_old = ...
    abs(omega_z)-abs(omega_opp_z);

d_omega_diff = ...
    (omega_diff-omega_diff_old)/Ts_eff;


alpha_diverge = ...
    (~startup_guard) && ...
    alpha_warn && ...
    (alpha_drv > ...
     alpha_opp_drv+alpha_diff_thr);


omega_diverge = ...
    (~startup_guard) && ...
    (omega_diff > omega_diff_thr) && ...
    (d_omega_diff > omega_diff_rate_thr);


axis_diverge = ...
    alpha_diverge || omega_diverge;


%% ============================================================
% 19. Normal状态进入条件
% =============================================================

risk_enter_raw = false;
warn_enter_raw = false;

if state_z == 0.0 && ...
        active && ...
        (~initial_blank)

    % 路径1：负载严重降低并伴随动态异常
    risk_path_main = ...
        load_low_risk && ...
        (alpha_risk || load_drop_risk);

    % 路径2：负载中度降低且快速恶化
    risk_path_dynamic = ...
        detector_armed && ...
        (q_full < q_dynamic_thr) && ...
        load_drop_risk && ...
        alpha_warn;

    % 路径3：极强角加速度且负载已经下降
    risk_path_strong = ...
        detector_armed && ...
        alpha_strong && ...
        (q_full < 0.90);

    % 路径4：持续严重负载不足
    % 不要求alpha必须明显异常
    risk_path_sustained_load = ...
        severe_load_confirmed;

    risk_enter_raw = ...
        risk_path_main || ...
        risk_path_dynamic || ...
        risk_path_strong || ...
        risk_path_sustained_load;


    % Warning：中度负载异常
    warn_path_main = ...
        load_low_warn && ...
        (alpha_warn || load_drop_warn);

    warn_enter_raw = ...
        warn_path_main;
end


% Risk优先
if risk_enter_raw
    warn_enter_raw = false;
end


%% ============================================================
% 20. Normal状态进入确认计数
% =============================================================

if risk_enter_raw

    risk_enter_cnt = risk_enter_cnt + 1.0;

    if risk_enter_cnt > risk_enter_steps
        risk_enter_cnt = risk_enter_steps;
    end

else

    risk_enter_cnt = 0.0;
end


if warn_enter_raw

    warn_enter_cnt = warn_enter_cnt + 1.0;

    if warn_enter_cnt > warn_enter_steps
        warn_enter_cnt = warn_enter_steps;
    end

else

    warn_enter_cnt = 0.0;
end


risk_enter = ...
    (risk_enter_cnt >= risk_enter_steps);

warn_enter = ...
    (warn_enter_cnt >= warn_enter_steps);


%% ============================================================
% 21. Warning重新升级Risk
%
% 满足任一条件：
%   1. 极强角加速度；
%   2. 持续严重负载能力不足；
%   3. 负载支持能力低且角加速度异常。
% =============================================================

risk_reenter_raw = ...
    (state_z == 1.0) && ...
    active && ...
    ( ...
      alpha_strong || ...
      severe_load_confirmed || ...
      ( ...
        (q_support < support_reenter_thr) && ...
        alpha_warn ...
      ) ...
    );


if risk_reenter_raw

    risk_reenter_cnt = risk_reenter_cnt + 1.0;

    if risk_reenter_cnt > risk_reenter_steps
        risk_reenter_cnt = risk_reenter_steps;
    end

else

    risk_reenter_cnt = 0.0;
end


risk_reenter = ...
    (risk_reenter_cnt >= risk_reenter_steps);


%% ============================================================
% 22. 三状态状态机
% =============================================================

if ~active

    % --------------------------------------------------------
    % 无驱动请求
    % --------------------------------------------------------

    state_z = 0.0;

    state_hold_cnt = 0.0;
    stable_cnt = 0.0;


elseif state_z == 0.0

    % --------------------------------------------------------
    % Normal
    % --------------------------------------------------------

    state_hold_cnt = 0.0;
    stable_cnt = 0.0;

    if risk_enter

        % 根据检测时负载能力确定Risk限扭比例
        ratio_candidate = ...
            q_full+risk_ratio_margin;

        if ratio_candidate < risk_ratio_min

            risk_ratio_z = risk_ratio_min;

        elseif ratio_candidate > risk_ratio_max

            risk_ratio_z = risk_ratio_max;

        else

            risk_ratio_z = ratio_candidate;
        end

        state_z = 2.0;

        risk_enter_cnt = 0.0;
        warn_enter_cnt = 0.0;
        risk_reenter_cnt = 0.0;
        severe_load_cnt = 0.0;

        state_hold_cnt = 0.0;
        stable_cnt = 0.0;


    elseif warn_enter

        state_z = 1.0;

        warn_enter_cnt = 0.0;
        risk_reenter_cnt = 0.0;

        state_hold_cnt = 0.0;
        stable_cnt = 0.0;
    end


elseif state_z == 2.0

    % --------------------------------------------------------
    % Risk：快速限扭
    % --------------------------------------------------------

    state_hold_cnt = state_hold_cnt + 1.0;

    if state_hold_cnt >= risk_hold_steps

        risk_stable = ...
            (q_support > support_risk_recover_thr) && ...
            (alpha_drv < 0.55*alpha_thr_eff);

        if risk_stable

            stable_cnt = stable_cnt + 1.0;

            if stable_cnt >= risk_stable_steps

                % Risk先退出到Warning
                state_z = 1.0;

                state_hold_cnt = 0.0;
                stable_cnt = 0.0;

                risk_reenter_cnt = 0.0;
                severe_load_cnt = 0.0;
            end

        else

            stable_cnt = 0.0;
        end
    end


else

    % --------------------------------------------------------
    % Warning：轻度限扭/恢复观察
    % --------------------------------------------------------

    state_hold_cnt = state_hold_cnt + 1.0;

    if risk_reenter

        % 重新恶化，根据当前执行比例再下降约10%
        ratio_candidate = ...
            torque_ratio_applied-0.10;

        if ratio_candidate < risk_ratio_min

            risk_ratio_z = risk_ratio_min;

        elseif ratio_candidate > risk_ratio_max

            risk_ratio_z = risk_ratio_max;

        else

            risk_ratio_z = ratio_candidate;
        end

        state_z = 2.0;

        state_hold_cnt = 0.0;
        stable_cnt = 0.0;

        risk_reenter_cnt = 0.0;
        severe_load_cnt = 0.0;


    elseif state_hold_cnt >= warn_hold_steps

        % Warning期间已经执行82%轻度限扭，
        % 因此不能再要求Te/Treq > 0.95，否则无法退出。
        normal_recovered = ...
            (q_support > support_normal_thr) && ...
            (abs(alpha_drv) < 0.40*alpha_thr_eff) && ...
            (~severe_load_confirmed);

        if normal_recovered

            stable_cnt = stable_cnt + 1.0;

            if stable_cnt >= warn_stable_steps

                state_z = 0.0;

                state_hold_cnt = 0.0;
                stable_cnt = 0.0;

                risk_reenter_cnt = 0.0;
                severe_load_cnt = 0.0;

                % 防止刚回Normal时恢复扭矩造成再次误触发
                cooldown_cnt = cooldown_steps;
            end

        else

            stable_cnt = 0.0;
        end
    end
end


%% ============================================================
% 23. 输出
% =============================================================

state = state_z;

risk = ...
    (state_z == 2.0);

warn = ...
    (state_z == 1.0);


if state_z == 2.0

    % Risk：自适应强限扭
    limit_ratio = risk_ratio_z;

elseif state_z == 1.0

    % Warning：82%轻度限扭
    limit_ratio = warning_limit_ratio;

else

    % Normal：不限制
    limit_ratio = 1.0;
end


%% ============================================================
% 24. 更新历史量
% =============================================================

omega_z = omega;
omega_opp_z = omega_opp;

% 当前版本保留对轴负载接口
unused_Tload_opp = Tload_opp; %#ok<NASGU>

end

== matlab function TPTC_Vehicle_dynamics_pedal2torque_NeglectSOC/Powertrain/03_MCU_TPTC_Controller/Command_Merge_Front/Fast_Down_Slow_Up_Limiter ==
  data: T_vcu_f input; T_cmd_f output; T_vcu_r input; Tlim_f input; Tlim_r input; T_damp_f input; T_damp_r input; T_cmd_r output
function [T_cmd_f, T_cmd_r] = f(T_vcu_f, T_vcu_r, Tlim_f, Tlim_r, T_damp_f, T_damp_r)
%#codegen

% Front axle
T_base_f = min(T_vcu_f, Tlim_f);
T_tmp_f = T_base_f + T_damp_f;

if T_tmp_f > Tlim_f
    T_cmd_f = Tlim_f;
elseif T_tmp_f < 0
    T_cmd_f = 0;
else
    T_cmd_f = T_tmp_f;
end

% Rear axle
T_base_r = min(T_vcu_r, Tlim_r);
T_tmp_r = T_base_r + T_damp_r;

if T_tmp_r > Tlim_r
    T_cmd_r = Tlim_r;
elseif T_tmp_r < 0
    T_cmd_r = 0;
else
    T_cmd_r = T_tmp_r;
end

end
